simulink model "thermal_noise"  (R2021b)
settings: Solver=VariableStepAuto  StartTime=0.0  StopTime=100.0  RelTol=1e-3
settings Model: Creator=DELL  LastModifiedBy=DELL

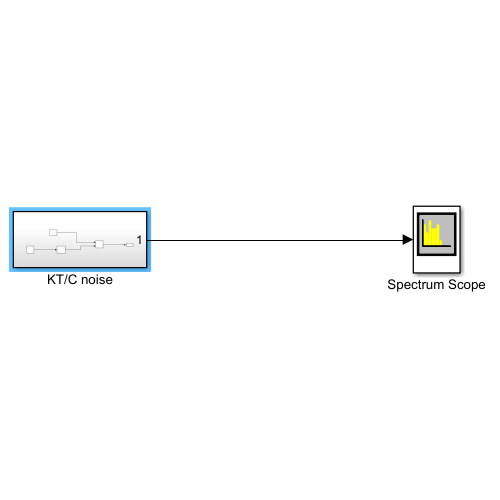
[thumbnail: Simulink's stored preview of the top-level diagram]
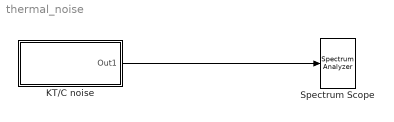
== system thermal_noise ==
  KT/C noise : Subsystem
  Spectrum Scope : SpectrumAnalyzer
  wires:
  KT/C noise/1(Out1) -> Spectrum Scope/1

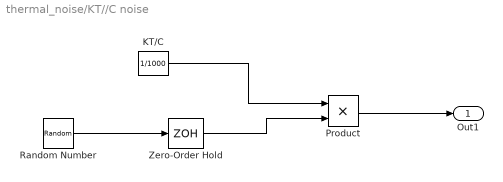
== system thermal_noise/KT//C noise ==
  KT/C : Constant  Value=1/1000
  Product : Product
  Random Number : RandomNumber  SampleTime=0.01
  Zero-Order Hold : ZeroOrderHold  SampleTime=-1
  Out1 : Outport
  wires:
  Random Number/1 -> Zero-Order Hold/1
  Zero-Order Hold/1 -> Product/2
  KT/C/1 -> Product/1
  Product/1 -> Out1/1
